simulink model "Lecture2_DC_Motor"  (R2020b)
settings: Solver=VariableStepAuto  StartTime=0.0  StopTime=10.0  RelTol=1e-3
settings Model: Creator=sebastian  LastModifiedBy=sebastian

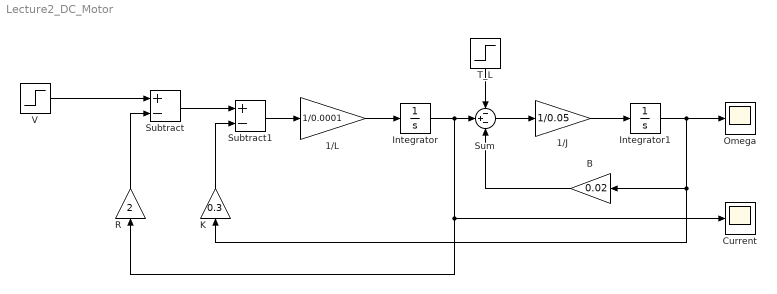
== system Lecture2_DC_Motor ==
  1/J : Gain  Gain=1/0.05
  1/L : Gain  Gain=1/0.0001
  B : Gain  Gain=0.02
  Current : Scope
  Integrator : Integrator
  Integrator1 : Integrator
  K : Gain  Gain=0.3
  Omega : Scope
  R : Gain  Gain=2
  Subtract : Sum  Inputs=+-
  Subtract1 : Sum  Inputs=+-
  Sum : Sum  Inputs=-+-
  T_L : Step  Time=5  After=2  SampleTime=0
  V : Step  After=10  SampleTime=0
  wires:
  V/1 -> Subtract/1
  R/1 -> Subtract/2
  K/1 -> Subtract1/2
  Subtract/1 -> Subtract1/1
  Subtract1/1 -> 1/L/1
  1/L/1 -> Integrator/1
  Integrator/1 -> Sum/2, Current/1, R/1
  T_L/1 -> Sum/1
  Sum/1 -> 1/J/1
  1/J/1 -> Integrator1/1
  Integrator1/1 -> Omega/1, B/1, K/1
  B/1 -> Sum/3
